simulink model "podB"  (R2024b)
settings: Solver=VariableStepAuto  StartTime=0.0  StopTime=10.0  RelTol=1e-3
settings Model: Creator=Ishak  LastModifiedBy=Ishak

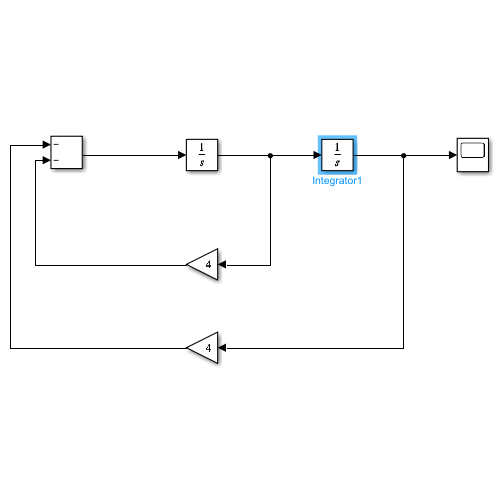
[thumbnail: Simulink's stored preview of the top-level diagram]
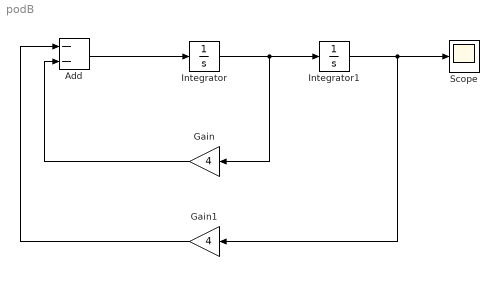
== system podB ==
  Add : Sum  Inputs=--
  Gain : Gain  Gain=4
  Gain1 : Gain  Gain=4
  Integrator : Integrator
  Integrator1 : Integrator  InitialCondition=1
  Scope : Scope
  wires:
  Add/1 -> Integrator/1
  Integrator/1 -> Gain/1, Integrator1/1
  Integrator1/1 -> Gain1/1, Scope/1
  Gain/1 -> Add/2
  Gain1/1 -> Add/1
